simulink model "regulator_2015a"  (R2015a)
settings: Solver=ode45  StartTime=0.0  StopTime=10.0  RelTol=1e-3
values from neighbouring files (symbols this model uses):
  Kp = 100    [matlab.mat]    (also in motor.m = 18.6)
  Td = 0.00117375026294    [matlab.mat]
  Ti = 0.068    [matlab.mat]
settings Model: CovExternalEMLEnable=on  Creator=thomakro  LastModifiedBy=ewilthil
settings DataIOCC: SignalLoggingSaveFormat=ModelDataLogs
settings OptimizationCC: InitFltsAndDblsToZero=on
settings DebuggingCC: SaveWithParameterizedLinksMsg=none  UnderspecifiedInitializationDetection=Classic  MergeDetectMultiDrivingBlocksExec=none  SignalResolutionControl=TryResolveAllWithWarning  SolverPrmCheckMsg=warning  FcnCallInpInsideContextMsg=EnableAllAsWarning
settings SFSimCC: SimUseLocalCustomCode=on
settings RTWCC: RTWUseLocalCustomCode=on
settings GRTTargetCC: TargetFcnLib=ansi_tfl_tmw.mat  GeneratePreprocessorConditionals=Use local settings  CombineOutputUpdateFcns=off  GRTInterface=on

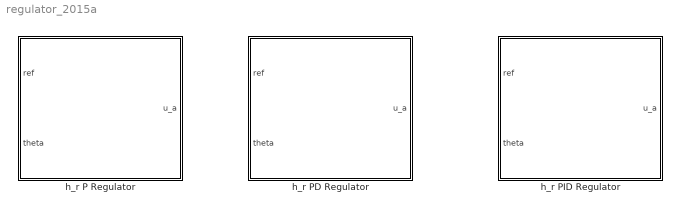
== system regulator_2015a ==
  h_r P Regulator : Subsystem  mask{Kp=Kp}
      mask Display:
      | image(imread('maxon_ctrl.jpg'))
      | port_label('input',1,'ref','texmode','on')
      | port_label('input',2,'\theta','texmode','on')
      | port_label('output',1,'u_a','texmode','on')
  h_r PD Regulator : Subsystem  mask{Kp=Kp, Td=Td}
      mask Display:
      | image(imread('maxon_ctrl.jpg'))
      | port_label('input',1,'ref','texmode','on')
      | port_label('input',2,'\theta','texmode','on')
      | port_label('output',1,'u_a','texmode','on')
  h_r PID Regulator : Subsystem  mask{Kp=Kp, Ti=Ti, Td=Td}
      mask Display:
      | image(imread('maxon_ctrl.jpg'))
      | port_label('input',1,'ref','texmode','on')
      | port_label('input',2,'\theta','texmode','on')
      | port_label('output',1,'u_a','texmode','on')

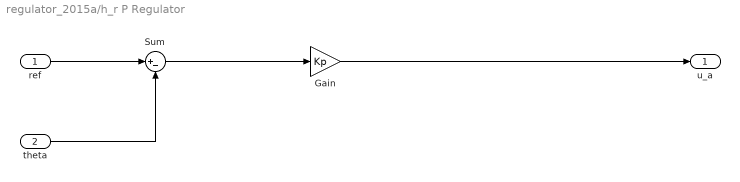
== system regulator_2015a/h_r P Regulator ==
  ref : Inport
  theta : Inport  Port=2
  Gain : Gain  Gain=Kp
  Sum : Sum  Inputs=|+-
  u_a : Outport
  wires:
  Gain/1 -> u_a/1
  ref/1 -> Sum/1
  theta/1 -> Sum/2
  Sum/1 -> Gain/1

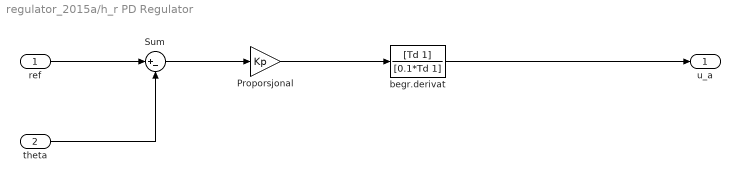
== system regulator_2015a/h_r PD Regulator ==
  ref : Inport
  theta : Inport  Port=2
  Proporsjonal : Gain  Gain=Kp
  Sum : Sum  Inputs=|+-
  begr.derivat : TransferFcn  Numerator=[Td 1]  Denominator=[0.1*Td 1]
  u_a : Outport
  wires:
  Sum/1 -> Proporsjonal/1
  theta/1 -> Sum/2
  ref/1 -> Sum/1
  begr.derivat/1 -> u_a/1
  Proporsjonal/1 -> begr.derivat/1

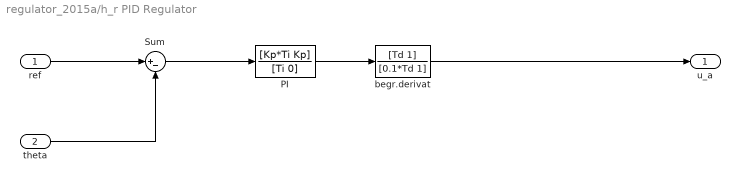
== system regulator_2015a/h_r PID Regulator ==
  ref : Inport
  theta : Inport  Port=2
  PI : TransferFcn  Numerator=[Kp*Ti Kp]  Denominator=[Ti 0]
  Sum : Sum  Inputs=|+-
  begr.derivat : TransferFcn  Numerator=[Td 1]  Denominator=[0.1*Td 1]
  u_a : Outport
  wires:
  PI/1 -> begr.derivat/1
  ref/1 -> Sum/1
  theta/1 -> Sum/2
  Sum/1 -> PI/1
  begr.derivat/1 -> u_a/1
